simulink model "mainController"  (R2019a)
settings: Solver=FixedStepDiscrete  StartTime=0  StopTime=inf  FixedStep=0.1  RelTol=1e-3
model workspace (MAT data in the model file):
  SL_ROS_VariableLengthArrays_MaxSizes : struct (value not decoded)
values from neighbouring files (symbols this model uses):
  numJoints = MotominiParams.numJoints    [showCompleteDemo.m]
  numPoints = size(Q,2)-2    [showCompleteDemo.m]
undefined symbols (not defined in the file or in its folder): homeToIdleSpline, idleToHomeSpline, objectSelect, Position, Position_SL_Info, Positions, Positions_SL_Info, TimeFromStart, userCommand, Velocities, Velocities_SL_Info
libraries: robotlib x19, visiontextngfix x6, simulink x2, visionsinks x2
(part 2 of 2)

== system mainController/Robot ROS Interfaces/Robot State/Get Finger Positions ==
  msg : Inport
  Enable : EnablePort
  Bus Selector : BusSelector  OutputSignals=Actual.Positions,Actual.Positions_SL_Info.CurrentLength
  Constant : Constant  Value=numJoints
  Data Type Conversion : DataTypeConversion  OutDataTypeStr=uint32
  Relational Operator : RelationalOperator  Operator===  OutDataTypeStr=boolean  RndMeth=Simplest
  Selector : Selector  InputPortWidth=16  IndexOptions=Index vector (dialog)  Indices=[1:numJoints]  OutputSizes=1
  gripperAct : Outport  InitialOutput=-1000*ones(numJoints,1)
  isValid : Outport  Port=2  InitialOutput=[0]
  wires:
  Relational Operator/1 -> isValid/1
  Data Type Conversion/1 -> Relational Operator/2
  Constant/1 -> Data Type Conversion/1
  Selector/1 -> gripperAct/1
  Bus Selector/2 -> Relational Operator/1  "<CurrentLength>"
  Bus Selector/1 -> Selector/1  "<Positions>"
  msg/1 -> Bus Selector/1

== system mainController/Robot ROS Interfaces/Robot State/Get Joint Positions ==
  msg : Inport
  Enable : EnablePort
  Bus Selector : BusSelector  OutputSignals=Actual.Positions,Actual.Positions_SL_Info.CurrentLength
  Constant : Constant  Value=numJoints
  Data Type Conversion : DataTypeConversion  OutDataTypeStr=uint32
  Relational Operator : RelationalOperator  Operator===  OutDataTypeStr=boolean  RndMeth=Simplest
  Selector : Selector  InputPortWidth=16  IndexOptions=Index vector (dialog)  Indices=[1:numJoints]  OutputSizes=1
  qAct : Outport  InitialOutput=-1000*ones(numJoints,1)
  isValid : Outport  Port=2  InitialOutput=[0]
  wires:
  msg/1 -> Bus Selector/1
  Bus Selector/1 -> Selector/1  "<Positions>"
  Bus Selector/2 -> Relational Operator/1  "<CurrentLength>"
  Selector/1 -> qAct/1
  Constant/1 -> Data Type Conversion/1
  Data Type Conversion/1 -> Relational Operator/2
  Relational Operator/1 -> isValid/1

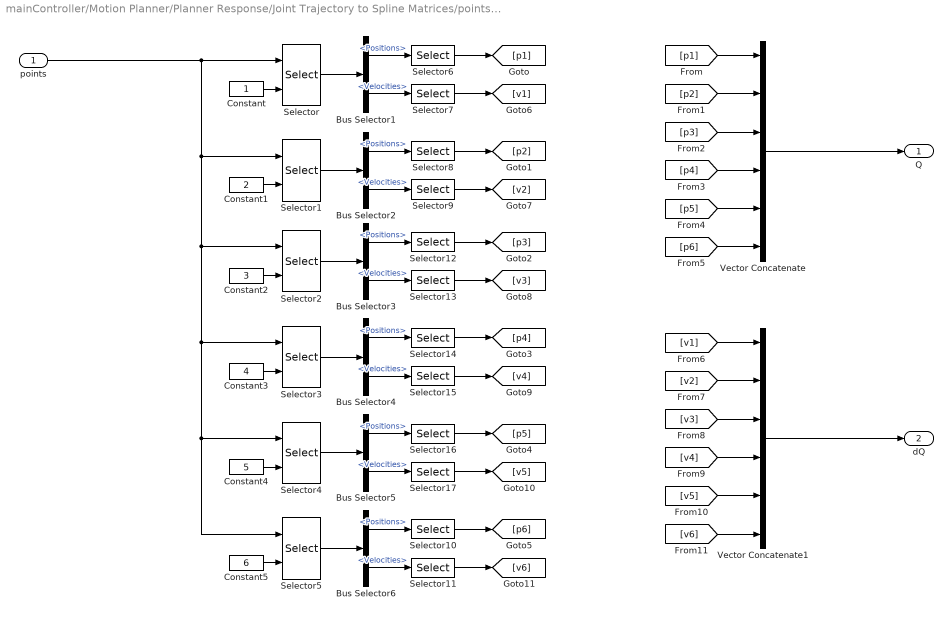
== system mainController/Motion Planner/Planner Response/Joint Trajectory to Spline Matrices/pointsToSplineWithBlocks ==
  points : Inport
  Bus Selector{1..6} (6 alike) : BusSelector  OutputSignals=Positions,Velocities
  Constant : Constant
  Constant1 : Constant  Value=2
  Constant2 : Constant  Value=3
  Constant3 : Constant  Value=4
  Constant4 : Constant  Value=5
  Constant5 : Constant  Value=6
  Selector{,1..5} (6 alike) : Selector  InputPortWidth=16  IndexOptions=Index vector (port)  Indices=[1]  OutputSizes=1
  Selector{6..17} (12 alike) : Selector  IndexOptions=Index vector (dialog)  Indices=[1:numJoints]  OutputSizes=1
  Vector Concatenate : Concatenate  NumInputs=6  Mode=Multidimensional array  ConcatenateDimension=2
  Vector Concatenate1 : Concatenate  NumInputs=6  Mode=Multidimensional array  ConcatenateDimension=2
  Q : Outport
  dQ : Outport  Port=2
  wires:
  [v4] -> Vector Concatenate1/4
  Constant1/1 -> Selector1/2
  Bus Selector5/1 -> Selector16/1  "<Positions>"
  Constant5/1 -> Selector5/2
  Bus Selector3/1 -> Selector12/1  "<Positions>"
  Selector4/1 -> Bus Selector5/1
  Vector Concatenate/1 -> Q/1
  Bus Selector3/2 -> Selector13/1  "<Velocities>"
  Bus Selector4/2 -> Selector15/1  "<Velocities>"
  Bus Selector1/1 -> Selector6/1  "<Positions>"
  Bus Selector2/2 -> Selector9/1  "<Velocities>"
  Selector/1 -> Bus Selector1/1
  points/1 -> Selector1/1, Selector2/1, Selector3/1, Selector4/1, Selector5/1, Selector/1
  Bus Selector6/2 -> Selector11/1  "<Velocities>"
  Selector1/1 -> Bus Selector2/1
  Constant/1 -> Selector/2
  Bus Selector5/2 -> Selector17/1  "<Velocities>"
  Selector3/1 -> Bus Selector4/1
  Selector5/1 -> Bus Selector6/1
  Selector2/1 -> Bus Selector3/1
  Bus Selector4/1 -> Selector14/1  "<Positions>"
  Bus Selector2/1 -> Selector8/1  "<Positions>"
  Constant3/1 -> Selector3/2
  Constant2/1 -> Selector2/2
  Bus Selector1/2 -> Selector7/1  "<Velocities>"
  Constant4/1 -> Selector4/2
  Bus Selector6/1 -> Selector10/1  "<Positions>"
  Selector6/1 -> [p1]
  Selector17/1 -> [v5]
  [v5] -> Vector Concatenate1/5
  Selector12/1 -> [p3]
  Selector8/1 -> [p2]
  Selector15/1 -> [v4]
  Selector14/1 -> [p4]
  Vector Concatenate1/1 -> dQ/1
  [v6] -> Vector Concatenate1/6
  [p4] -> Vector Concatenate/4
  [v3] -> Vector Concatenate1/3
  Selector16/1 -> [p5]
  [p3] -> Vector Concatenate/3
  Selector9/1 -> [v2]
  [p6] -> Vector Concatenate/6
  Selector13/1 -> [v3]
  [p1] -> Vector Concatenate/1
  Selector7/1 -> [v1]
  [v1] -> Vector Concatenate1/1
  [p2] -> Vector Concatenate/2
  [v2] -> Vector Concatenate1/2
  Selector11/1 -> [v6]
  [p5] -> Vector Concatenate/5
  Selector10/1 -> [p6]

== stateflow chart mainController/Speech Command Recognizer/Enabled Subsystem/Chart ==
  state Idle
    en:
    userCommand=0;
    objectSelect=1;
  state Object_Selecting
    en:
    objectSelect = 1*(voiceCommand=="left") ...
    + 2*(voiceCommand=="right") ...
    + 3*(voiceCommand=="forward");
  state Start_Grasping
    en:
    userCommand=1;
  (default) -> Idle
  Idle -> Object_Selecting : [hasData && voiceCommand != "go"&&voiceCommand != "stop"]
  Object_Selecting -> Idle [order 1] : [hasData && voiceCommand=="stop"]
  Start_Grasping -> Idle : [isHome]
  Object_Selecting -> Start_Grasping [order 2] : [hasData && voiceCommand=="go"]
  data: voiceCommand input; objectSelect output; userCommand output; isHome input; hasData input

== matlab function mainController/Motion Planner/Planner Response/Joint Trajectory to Spline Matrices/pointsToSplineData ==
  data: pointsMsg input; Q output double size=[numJoints, numPoints+2]; dQ output double size=[numJoints, numPoints+2]; t output double size=[1, numPoints+2]; numJoints parameter; numPoints parameter; isValid output boolean size=[1]
function [Q,dQ,t, isValid] = pointsMsgToSplineData(pointsMsg,numJoints,numPoints)
% Author: Carlos Santacruz-Rosero, Ph.D.
% Copyright 2016 The MathWorks, Inc.

points = pointsMsg(1:numPoints+2);

Q = zeros(numJoints, numPoints+2);
dQ = zeros(numJoints, numPoints+2);
t = zeros(1,numPoints+2);
isValid = true;

numRxJoints = points(1).Positions_SL_Info.CurrentLength;

if numRxJoints ~= numJoints
    isValid = false;
end

for ii = 1:(numPoints+2)
    Q(:,ii) = points(ii).Positions(1:numJoints);
    dQ(:,ii) = points(ii).Velocities(1:numJoints);
    dur = points(ii).TimeFromStart;
    t(ii) =  double(dur.Sec)+double(dur.Nsec)*10^-9;
end

== stateflow chart mainController/State Controller/State Controller ==
  state Home
    state Home
      entry:
      requestTrajController = false;
      requestGripController = false;
      plannerRequest= false;
      droppingPos = [-0.1;0.2;0.1];
      gripperOpenPos = [0.050; 0.050];
      gripperClosedPos =[0; 0];
      isHome = true;
    state GoingToHome
      entry:
      % move arm
      requestTrajController = true;
      Qspline = idleToHomeSpline.Q;
      dQspline = idleToHomeSpline.dQ;
      tSpline = idleToHomeSpline.t;
      goalSpline = idleToHomeSpline.Q(:,end);
      % close gripper
      requestGripController = true;
      gripCommand = [0; 0];
      during: % Going To Target
      requestTrajController = false;
      requestGripController = false;
    (default) -> Home.Home
    (junction 80) -> Home.Home
    GoingToHome -> (junction 80) : [goalReached && qActIsValid]
  state Idle
    state GoingToIdle
      entry:
      % move arm
      requestTrajController = true;
      Qspline = homeToIdleSpline.Q;
      dQspline = homeToIdleSpline.dQ;
      tSpline = homeToIdleSpline.t;
      goalSpline = homeToIdleSpline.Q(:,end);
      % open gripper
      requestGripController = true;
      gripCommand = gripperOpenPos;
      during: % Going To Target
      requestTrajController = false;
      requestGripController = false;
    state Idle
      entry:
      objectDetected = uint32(0);
      objectDetectedPos = zeros(3,1);
      % open gripper
      requestGripController = true;
      gripCommand = gripperOpenPos;
      isHome = false;
      during:
      [objectDetected, objectDetectedPos,droppingPos] = isObjectInScene(detectorPredictedLabels, detectorXYZPoints,objectSelect)
      requestGripController = false;
    GoingToIdle -> Idle.Idle : [goalReached && qActIsValid]
  state Grabbing
    state RequestGrabbingPlan
      entry:
      plannerRequest= true;
      requestTrajController=false;
      plannerObjectID = objectDetected;
      plannerPos = [objectDetectedPos(1);
      objectDetectedPos(2);
      objectDetectedPos(3)+0.01];
      during:
      plannerRequest= false;
      exit:
    state GoingToApproachPoint
      entry:
      requestTrajController = true;
      Qspline = plannerQ;
      dQspline = plannerDQ;
      tSpline = plannerT;
      goalSpline = plannerQ(:,end);
      during: % Going To Target
      requestTrajController = false;
    state RequestApproachingPlan
      entry:
      plannerRequest= true;
      plannerObjectID = objectDetected;
      plannerPos = [objectDetectedPos(1);
      objectDetectedPos(2);
      objectDetectedPos(3)+0.1];
      during:
      plannerRequest= false;
    state DroppingObject
      entry:
      requestGripController = true;
      gripCommand = gripperOpenPos;
      during: % Going To Target
      requestGripController = false;
    state GoingToObject
      entry:
      requestTrajController = true;
      Qspline = plannerQ;
      dQspline = plannerDQ;
      tSpline = plannerT;
      goalSpline = plannerQ(:,end);
      during: % Going To Target
      requestTrajController = false;
    state RequestLeavingPlan
      entry:
      plannerRequest= true;
      plannerObjectID = objectDetected;
      plannerPos = [objectDetectedPos(1);
      objectDetectedPos(2);
      objectDetectedPos(3)+0.1];
      during:
      plannerRequest= false;
      exit:
    state GrabbingObject
      entry:
      gripCommand = gripperClosedPos;
      requestGripController = true;
      during: % Going To Target
      requestGripController = false;
    state GoingToLeavingPoint
      entry:
      requestTrajController = true;
      Qspline = plannerQ;
      dQspline = plannerDQ;
      tSpline = plannerT;
      goalSpline = plannerQ(:,end);
      during: % Going To Leaving Point
      requestTrajController = false;
    state GoingToDroppingPoint
      entry:
      requestTrajController = true;
      Qspline = plannerQ;
      dQspline = plannerDQ;
      tSpline = plannerT;
      goalSpline = plannerQ(:,end);
      during: % Going To Target
      requestTrajController = false;
    state RequestDroppingPlan
      entry:
      plannerRequest= true;
      plannerObjectID = objectDetected;
      plannerPos = droppingPos;
      during:
      plannerRequest= false;
    RequestGrabbingPlan -> GoingToObject : [plannerHasReplied && ...
        | plannerIsValid]
    RequestApproachingPlan -> GoingToApproachPoint : [plannerHasReplied && ...
        | plannerIsValid]
    GoingToApproachPoint -> RequestGrabbingPlan : [goalReached && qActIsValid]
    GoingToDroppingPoint -> DroppingObject : [goalReached && qActIsValid]
    GoingToObject -> GrabbingObject : [goalReached && qActIsValid]
    GrabbingObject -> RequestLeavingPlan : [~isGripperOpen]
    RequestLeavingPlan -> GoingToLeavingPoint : [plannerHasReplied && ...
        | plannerIsValid]
    RequestDroppingPlan -> GoingToDroppingPoint : [plannerHasReplied && ...
        | plannerIsValid]
    GoingToLeavingPoint -> RequestDroppingPlan : [goalReached && qActIsValid]
  Home.Home -> Idle.Idle : [armCommand==1]
  (default) -> Home
  DroppingObject -> GoingToIdle : [isGripperOpen]
  Idle.Idle -> GoingToHome [order 1] : [(~requestGripController&&objectSelect~=0&&objectDetected==0)||objectSelect==0]
  Idle.Idle -> RequestApproachingPlan [order 2] : [(objectDetected ~=0) && qActIsValid]
  data: objDetected function_output uint32; objPos function_output; labels function_input uint32; points function_input double; dropPos function_output; objSelect function_input; armCommand input uint32; objectSelect input; detectorPredictedLabels input uint32 size=[10 1]; detectorXYZPoints input double size=[10 3]; plannerHasReplied input boolean size=[1]; plannerQ input double; plannerDQ input double; plannerT input double; plannerIsValid input boolean; qActIsValid input boolean; plannerRequest output boolean size=[1]; plannerPos output double size=[3]; plannerObjectID output uint32 size=[1]; requestTrajController output boolean size=[1]; Qspline output double; dQspline output double; tSpline output; goalReached input boolean; homeToIdleSpline parameter; idleToHomeSpline parameter; requestGripController output boolean; gripCommand output double size=[2 1]; goalSpline output double size=[numJoints,1] =zeros(numJoints,1); gripperOpenPos local =[0.025;0.025]; gripperClosedPos local =[0;0]; droppingPos local; objectDetected local uint32 size=[1]; objectDetectedPos local double size=[3]; data1 local; isGripperOpen input; isHome output
  function [objDetected,objPos,dropPos] = isObjectInScene(labels, points, objSelect):
    | function [objDetected,objPos,dropPos] = isObjectInScene(labels, points, objSelect)
    | 
    | objDetected = uint32(0);
    | objPos = zeros(3,1);
    | dropPositions = [-0.20 0.2 0.1; -0.10 0.2 0.1; 0.00 0.2 0.1];
    | dropPos = zeros(3,1);
    | 
    | if ~isempty(labels)
    |     if objSelect==0
    |         objDetected = labels(1);
    |         objPos(1:3,1) = points(1,:)';
    |         objPos(1,1) = objPos(1,1) - 0.01;
    |         dropPos = dropPositions(objDetected,:)';
    |     else
    |         maxLabels = length(labels);
    |         for ii =1:maxLabels
    |             if objSelect == labels(ii)
    |                 objDetected = labels(ii);
    |                 objPos(1:3,1) = points(ii,:)';
    |                 dropPos = dropPositions(objDetected,:)';
    |                 return;
    |             end
    |         end
    |     end
    | end

== matlab function mainController/YOLO v2 Object Detector & Pose Estimator/Display/AddLabel ==
  data: image_raw input; image_label output; bboxes input size=[10 4]; labelsID input size=[1 3]
function image_label = addLabeltoImage(image_raw, bboxes, labelsID)
ARM_ID = 1;
DISK_ID = 2;
BRACE_ID = 3;

% 色付け表示
object_num = numel(labelsID);
cmaps = im2uint8(jet(3));
cmaps2=[cmaps(1,1) cmaps(1,2) cmaps(1,3);
       cmaps(3,1) cmaps(3,2) cmaps(3,3);
       cmaps(2,1) cmaps(2,2) cmaps(2,3)];
image_label = image_raw;

for k = 1: object_num
    label_str = 'unknown';
    if labelsID(k) == ARM_ID
        label_str = 'arm_part';
    elseif labelsID(k) == DISK_ID
        label_str = 'disk_part';
    elseif labelsID(k) == BRACE_ID
        label_str = 't_brace_part';
    end

    cmaps_tmp = [cmaps2(labelsID(k),1) cmaps2(labelsID(k),2) cmaps2(labelsID(k),3)];
    %labelStr = LABEL_STR(labelsID(k));
    if ~isempty(bboxes)
        image_label = insertObjectAnnotation(image_label,'rectangle',...
            bboxes(k,:),label_str,'Color',cmaps_tmp,'FontSize',20);
    end
    %figure, imshow(image_label);
end

== matlab function mainController/YOLO v2 Object Detector & Pose Estimator/Display/MATLAB Function1 ==
  data: u input size=[1 3]; y output size=[1 3]
function y = genSequence(u) %#codegen
     z = int32(find(u));
     y_tmp = size(z);
     for k=1:numel(y_tmp)
         y_tmp(k) = u(z(k));
     end
     
     y=int32(y_tmp);
%    y = int32(find(u));

== matlab function mainController/YOLO v2 Object Detector & Pose Estimator/Display/Formatting ==
  data: predictedLabels input size=[10 1]; Variables output size=[5 10]; xyzPoints input size=[10 3]; Color output size=[10 3]; Location output size=[10 2]
function [Variables,Color,Location] = concatenateVectors(predictedLabels,xyzPoints)
%#codegen
    Variables = single([1:size(predictedLabels,1); predictedLabels'; xyzPoints']);
    Color = ones(size(predictedLabels,1),3,'single');
    Location = [zeros(size(predictedLabels,1),1,'single') single((0:(size(predictedLabels,1)-1))'*25)];

== matlab function mainController/YOLO v2 Object Detector & Pose Estimator/Display/MATLAB Function ==
  data: u input size=[10 1]; y output size=[10 1]
function y = genSequence(u) %#codegen
    y = int32(find(u));

== matlab function mainController/Robot ROS Interfaces/Arm Trajectory Controller/ Assign Joint Trajectory ==
  data: blankMessage input; jointTrajPoints input; msg output Bus: SL_Bus_mainController_trajectory_msgs_JointTrajectory
function msg = assignJointTrajectory(blankMessage, jointTrajPoints)
%#codegen

% To set datatype of MSG output:
%  1. Create buses for this model: robotics.ros.createSimulinkBus(gcs)
%  1. Click "Edit Data" in  Toolstrip to open "Ports and Data Manager"
%  2. Select MSG and set datatype to "Bus: SL_Bus_<modelname>_<messageType>"
% See:
% http://www.mathworks.com/help/simulink/ug/create-structures-in-matlab-function-blocks.html


% Assign string array with joint names:
strArrayToAssign = {'joint_1_s',...
    'joint_2_l',...
    'joint_3_u',...
    'joint_4_r',...
    'joint_5_b',...
    'joint_6_t'};

% Assign Joint Trajectory Point:
numPoints = size(jointTrajPoints,1);
blankMessage.Points_SL_Info.CurrentLength = uint32(numPoints);
for ii = 1:numPoints
    blankMessage.Points(ii) = jointTrajPoints(ii);
end

numStringsInArray = length(strArrayToAssign);
blankMessage.JointNames_SL_Info.CurrentLength = uint32(numStringsInArray);

for idx=1:numStringsInArray
    str = strArrayToAssign{idx};
    strLength = length(str);
    blankMessage.JointNames(idx).Data(1:strLength) = uint8(str);
    blankMessage.JointNames(idx).Data_SL_Info.CurrentLength = uint32(strLength);
end

msg = blankMessage;

== matlab function mainController/Robot ROS Interfaces/Gripper Trajectory Controller/ Assign Joint Trajectory ==
  data: blankMessage input; jointTrajPoints input; msg output Bus: SL_Bus_mainController_trajectory_msgs_JointTrajectory
function msg = assignJointTrajectory(blankMessage, jointTrajPoints)
%#codegen

% To set datatype of MSG output:
%  1. Create buses for this model: robotics.ros.createSimulinkBus(gcs)
%  1. Click "Edit Data" in  Toolstrip to open "Ports and Data Manager"
%  2. Select MSG and set datatype to "Bus: SL_Bus_<modelname>_<messageType>"
% See: 
% http://www.mathworks.com/help/simulink/ug/create-structures-in-matlab-function-blocks.html


% Assign string array with joint names:
strArrayToAssign = {'gripper_finger_joint_l'; 'gripper_finger_joint_r'};

% Assign Joint Trajectory Point:
numPoints = size(jointTrajPoints,1);
blankMessage.Points_SL_Info.CurrentLength = uint32(numPoints);
for ii = 1:numPoints
    blankMessage.Points(ii) = jointTrajPoints(ii);
end

numStringsInArray = length(strArrayToAssign);
blankMessage.JointNames_SL_Info.CurrentLength = uint32(numStringsInArray);

for idx=1:numStringsInArray
    str = strArrayToAssign{idx};
    strLength = length(str);
    blankMessage.JointNames(idx).Data(1:strLength) = uint8(str);
    blankMessage.JointNames(idx).Data_SL_Info.CurrentLength = uint32(strLength);
end

msg = blankMessage;

== matlab function mainController/YOLO v2 Object Detector & Pose Estimator/Display/Formatting1 ==
  data: labelsID input size=[10 1]; Variables output size=[5 10]; xyzPoints input size=[10 3]; Color output size=[10 3]; Location output size=[10 2]
function [Variables,Color,Location] = concatenateVectors(labelsID,xyzPoints)
    Variables = single([1:size(labelsID,1); labelsID'; xyzPoints']);
    Color = ones(size(labelsID,1),3,'single');
    Location = [zeros(size(labelsID,1),1,'single') single((0:(size(labelsID,1)-1))'*25)];

== matlab function mainController/YOLO v2 Object Detector & Pose Estimator/Display/MATLAB Function2 ==
  data: u input size=[1 3]; y output size=[1 3]
function y = genSequence(u) %#codegen
     z = int32(find(u));
     y_tmp = z;
     for k=1:numel(y_tmp)
         y_tmp(k) = u(z(k));
     end
     
     y=int32(y_tmp);
%    y = int32(find(u));
